simulink model "observe_bldc"  (R2020a)
settings: Solver=FixedStepDiscrete  StartTime=0.0  StopTime=10  FixedStep=50e-6  RelTol=1e-3
undefined symbols (not defined in the file): sigbuilder_block
libraries: nesl_utility x12, ee_lib x9, fl_lib x6, simulink x2
settings Model: Creator=Tinh_deptrai  LastModifiedBy=Tinh_deptrai
settings SolverCC: AlgebraicLoopSolver=LineSearch

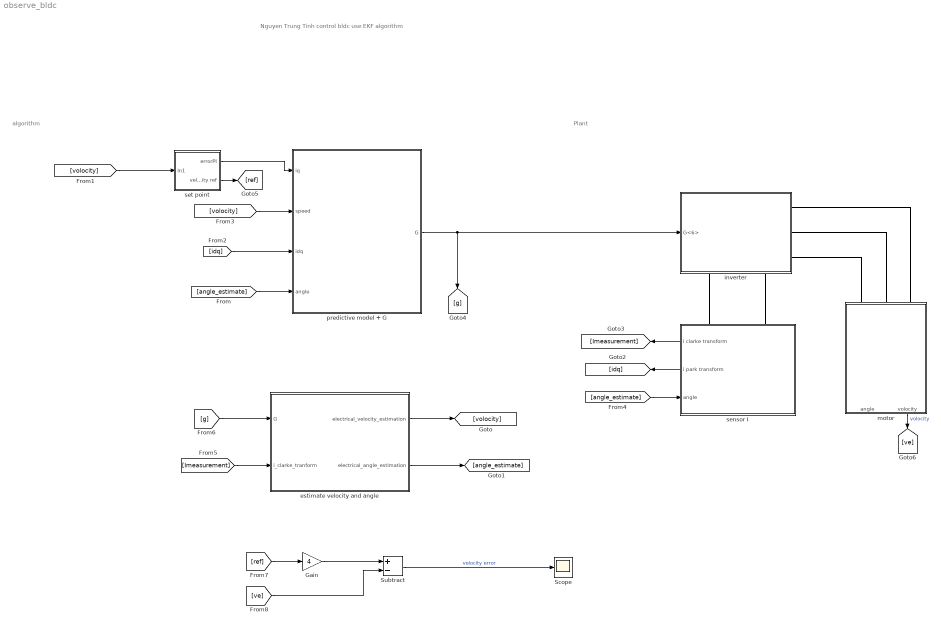
== system observe_bldc ==
  note: algorithm
  note: Nguyen Trung Tinh
      | control bldc use EKF algorithm
  note: Plant
  Gain : Gain  Gain=4
  Scope : Scope
  Subtract : Sum  Inputs=+-
  estimate velocity and angle : Subsystem
  inverter : Subsystem
      settings: PortSchema="{\"entries\":[{\"content\":{\"sides\":[{\"content\":{\"connectorIds\":[\"In1\"]},\"type\":\"ConnectorPlacement.EquallySpacedRectSide\",\"uuid\":\"9f8e1654-e76f-4ccd-87ff-712360a9448c\"},{\"content\":{\"connectorIds\":[\"RConn1\",\"RConn2\",\"RConn3\"],\"side\":\"RIGHT\"},\"type\":\"ConnectorPlacement.EquallySpacedRectSide\",\"uuid\":\"1603b82b-d8dc-4962-8b2e-607a69af6851\"},{\"content\":{\"connectorIds\":[],\"side\":\"TOP\"},\"type\":\"ConnectorPlacement.EquallySpacedRectSide\",\"uuid\":\"a55eb90c-eada-4bfc-8f9e-d2c70cbe25bd\"},{\"content\":{\"connectorIds\":[\"RConn4\",\"RConn5\"],\"side\":\"BOTTOM\"},\"type\":\"ConnectorPlacement.EquallySpacedRectSide\",\"uuid\":\"5facc57d-ea89-4f5b-8b06-1001d422b94e\"}]},\"type\":\"ConnectorPlacement.EquallySpacedConnector\",\"uuid\":\"acd0f578-42d7-4dc3-aef0-1ec9509de6cd\"}],\"packageUris\":[\"http://schema.mathworks.com/mf0/Connector/19700101\"],\"version\":\"1.0\"}"
  motor : Subsystem
  predictive model + G : Subsystem
  sensor I : Subsystem
      settings: PortSchema="{\"entries\":[{\"content\":{\"sides\":[{\"content\":{\"connectorIds\":[]},\"type\":\"ConnectorPlacement.EquallySpacedRectSide\",\"uuid\":\"0a592258-b95b-4330-8c63-2a9e4347ecac\"},{\"content\":{\"connectorIds\":[\"Out1\",\"Out2\",\"In1\"],\"side\":\"RIGHT\"},\"type\":\"ConnectorPlacement.EquallySpacedRectSide\",\"uuid\":\"44663962-0eca-4dc4-9145-5c0dbec9ec3a\"},{\"content\":{\"connectorIds\":[\"LConn1\",\"LConn2\"],\"side\":\"TOP\"},\"type\":\"ConnectorPlacement.EquallySpacedRectSide\",\"uuid\":\"ad629d0d-eb0f-4771-8bbd-1df9727b2b70\"}]},\"type\":\"ConnectorPlacement.EquallySpacedConnector\",\"uuid\":\"befa916a-8a4b-411d-a992-da4f8df3c86c\"}],\"packageUris\":[\"http://schema.mathworks.com/mf0/Connector/19700101\"],\"version\":\"1.0\"}"
  set point : Subsystem
  wires:
  [volocity] -> set point/1(In1)
  sensor I/1(" i clarke transform") -> [Imeasurement]
  sensor I/2(i park transform) -> [idq]
  set point/1(errorPI) -> predictive model + G/1(iq)
  [idq] -> predictive model + G/3(idq)
  [g] -> estimate velocity and angle/1(G)
  [Imeasurement] -> estimate velocity and angle/2(i_clarke_tranform)
  [angle_estimate] -> predictive model + G/4(angle)
  [volocity] -> predictive model + G/2(speed)
  [angle_estimate] -> sensor I/1(angle)
  predictive model + G/1(G) -> inverter/1(G<6>), [g]
  estimate velocity and angle/1(electrical_velocity_estimation) -> [volocity]
  estimate velocity and angle/2(electrical_angle_estimation) -> [angle_estimate]
  set point/2(velocity ref) -> [ref]
  [ref] -> Gain/1
  motor/2(volocity) -> [ve]  "volocity"
  [ve] -> Subtract/2
  Subtract/1 -> Scope/1  "velocity error"
  Gain/1 -> Subtract/1
  connections:
  motor/LConn1 -- inverter/RConn3
  motor/LConn2 -- inverter/RConn2
  motor/LConn3 -- inverter/RConn1
  sensor I/LConn2 -- inverter/RConn4
  sensor I/LConn1 -- inverter/RConn5

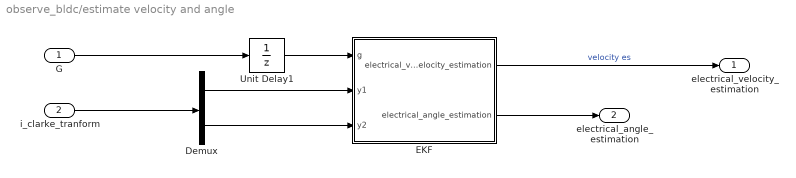
== system observe_bldc/estimate velocity and angle ==
  G : Inport
  i_clarke_tranform : Inport  Port=2
  Demux : Demux  Outputs=2
  EKF : Subsystem
  Unit Delay1 : UnitDelay  InitialCondition=1  SampleTime=-1  HasFrameUpgradeWarning=on
  electrical_velocity_estimation : Outport
  electrical_angle_estimation : Outport  Port=2
  wires:
  EKF/2(electrical_angle_estimation) -> electrical_angle_estimation/1
  Unit Delay1/1 -> EKF/1(g)
  i_clarke_tranform/1 -> Demux/1
  G/1 -> Unit Delay1/1
  Demux/1 -> EKF/2(y1)
  Demux/2 -> EKF/3(y2)
  EKF/1(electrical_velocity_estimation) -> electrical_velocity_estimation/1  "velocity es"

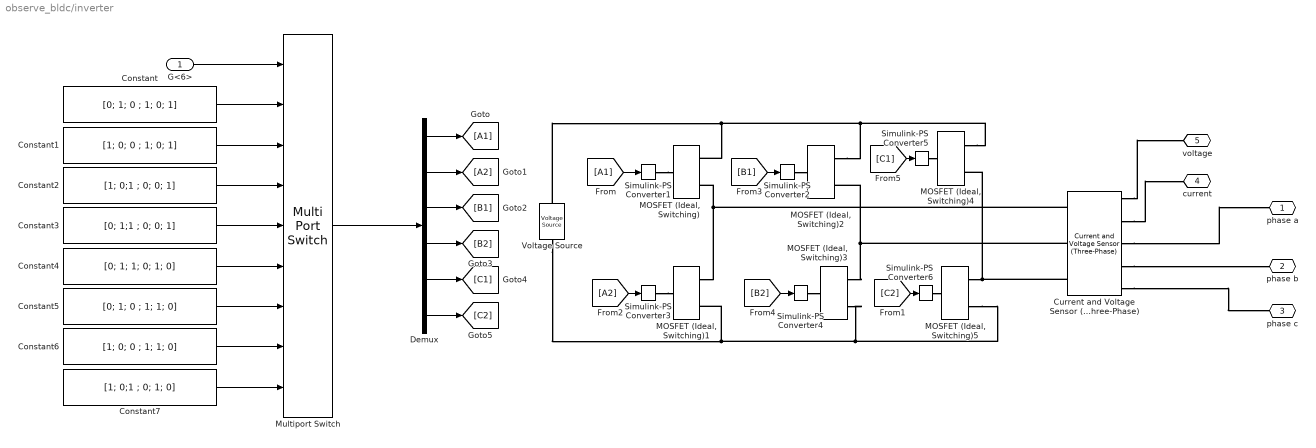
== system observe_bldc/inverter ==
  G<6> : Inport
  Constant : Constant  Value=[0; 1; 0 ; 1; 0; 1]
  Constant1 : Constant  Value=[1; 0; 0 ; 1; 0; 1]
  Constant2 : Constant  Value=[1; 0;1 ; 0; 0; 1]
  Constant3 : Constant  Value=[0; 1;1 ; 0; 0; 1]
  Constant4 : Constant  Value=[0; 1; 1; 0; 1; 0]
  Constant5 : Constant  Value=[0; 1; 0 ; 1; 1; 0]
  Constant6 : Constant  Value=[1; 0; 0 ; 1; 1; 0]
  Constant7 : Constant  Value=[1; 0;1 ; 0; 1; 0]
  Current and Voltage Sensor (Three-Phase) : ee_lib/Sensors & Transducers/Current and Voltage Sensor (Three-Phase)  vMeasurementType=ee.enum.vmeasurement.lg  outputUnit=ee.enum.unit.si  SRated=100e6 V*A  VRated=24e3 V  I_specify=off  I_priority=None  I=[ 0 0 0 ] A  I_nominal_specify=off  I_nominal_unit=A  I_nominal_value=1  V_specify=off  V_priority=None  V=[ 0 0 0 ] V  V_nominal_specify=off  V_nominal_unit=V  V_nominal_value=1
      settings: SourceProductBaseCode=PS  InternalSimscapePortConfiguration="{\"Bottom\":[],\"Left\":[{\"id\":\"a1\",\"label\":\"a1\",\"type\":\"foundation.electrical.electrical\"},{\"id\":\"b1\",\"label\":\"b1\",\"type\":\"foundation.electrical.electrical\"},{\"id\":\"c1\",\"label\":\"c1\",\"type\":\"foundation.electrical.electrical\"}],\"Right\":[{\"id\":\"V_output\",\"label\":\"V\",\"type\":\"output\"},{\"id\":\"I_output\",\"label\":\"I\",\"type\":\"output\"},{\"id\":\"a2\",\"label\":\"a2\",\"type\":\"foundation.electrical.electrical\"},{\"id\":\"b2\",\"label\":\"b2\",\"type\":\"foundation.electrical.electrical\"},{\"id\":\"c2\",\"label\":\"c2\",\"type\":\"foundation.electrical.electrical\"}],\"Top\":[]}"
  Demux : Demux  Outputs=6
  MOSFET (Ideal, Switching){,1..5} (6 alike) : ee_lib/Semiconductors & Converters/MOSFET (Ideal, Switching)  Rds=0.01 Ohm  Goff=1e-6 1/Ohm  Vth=0.5 V  diode_param=1  diode_Vf=0.8 V  diode_Ron=0.001 Ohm  diode_Goff=1e-5 1/Ohm  diode_C=50e-9 F  diode_iRM=-235 A  diode_iF=300 A  diode_idot=-50 A/us  diode_trr_param=1  diode_trr_factor=3  diode_trr=15 us  diode_Qrr=1500 s*uA  thermal_loss_option=2  Voff=300 V  Tau=1e-4 s  Tj=[298.15, 398.15] K  Iout_scalar=600 A  Eon_scalar=22.86e-3 J  Eoff_scalar=17.14e-3 J  Von_scalar=2.7 V  Iout_data=[0, 10, 50, 100, 200, 400, 600] A  Eon_data=[0, .29, 1.43, 2.86, 5.71, 13.14, 22.86; 0, .57, 2.63, 5.14, 10.29, 20.57, 30.29] * 1e-3 J  Eoff_data=[0, .21, 1.07, 2.14, 4.29, 9.86, 17.14; 0, .43, 1.97, 3.86, 7.71, 15.43, 22.71] * 1e-3 J  Von_data=[0, 1.1, 1.3, 1.45, 1.75, 2.25, 2.7; 0, 1, 1.15, 1.35, 1.7, 2.35, 3] V
  Multiport Switch : MultiPortSwitch  Inputs=8
  Simulink-PS Converter{1..6} (6 alike) : nesl_utility/Simulink-PS Converter  PhysicalDomain=network_engine_domain  SubClassName=ps_input  LeftPortType=input  RightPortType=output  PseudoPeriodic=off  Frequencies=[]  NoiseDistribution=none  NoiseParameters=[]  Unit=1  AffineConversion=off  FilteringAndDerivatives=provide  SimscapeFilterOrder=1  InputFilterTimeConstant=0.001  UdotUserProvided=0
  Voltage Source : ee_lib/Sources/Voltage Source  dc_voltage=48 V  ac_voltage=0 V  ac_shift=0 rad  ac_frequency=0 Hz  noise_mode=0  PSD=0 V^2/Hz  repeatability=1  auto_seed=4120125298  user_seed=0  sample_time=1e-3 s  i_specify=off  i_priority=None  i=0 A  i_nominal_specify=off  i_nominal_unit=A  i_nominal_value=1  v_specify=off  v_priority=None  v=0 V  v_nominal_specify=off  v_nominal_unit=V  v_nominal_value=1
  phase a : PMIOPort  Side=Right
  phase b : PMIOPort  Port=2  Side=Right
  phase c : PMIOPort  Port=3  Side=Right
  current : PMIOPort  Port=4  Side=Right
  voltage : PMIOPort  Port=5  Side=Right
  wires:
  Demux/4 -> [B2]
  Demux/1 -> [A1]
  [C2] -> Simulink-PS Converter6/1
  [A1] -> Simulink-PS Converter1/1
  Demux/3 -> [B1]
  [B1] -> Simulink-PS Converter2/1
  Demux/5 -> [C1]
  [A2] -> Simulink-PS Converter3/1
  Demux/2 -> [A2]
  Demux/6 -> [C2]
  [C1] -> Simulink-PS Converter5/1
  [B2] -> Simulink-PS Converter4/1
  G<6>/1 -> Multiport Switch/1
  Multiport Switch/1 -> Demux/1
  Constant/1 -> Multiport Switch/2
  Constant1/1 -> Multiport Switch/3
  Constant2/1 -> Multiport Switch/4
  Constant3/1 -> Multiport Switch/5
  Constant4/1 -> Multiport Switch/6
  Constant5/1 -> Multiport Switch/7
  Constant6/1 -> Multiport Switch/8
  Constant7/1 -> Multiport Switch/9
  connections:
  Voltage Source/RConn1 -- "MOSFET (Ideal, Switching)5"/RConn2 -- "MOSFET (Ideal, Switching)3"/RConn2 -- "MOSFET (Ideal, Switching)1"/RConn2
  Simulink-PS Converter5/RConn1 -- "MOSFET (Ideal, Switching)4"/LConn1
  Voltage Source/LConn1 -- "MOSFET (Ideal, Switching)4"/RConn1 -- "MOSFET (Ideal, Switching)2"/RConn1 -- "MOSFET (Ideal, Switching)"/RConn1
  Simulink-PS Converter2/RConn1 -- "MOSFET (Ideal, Switching)2"/LConn1
  "MOSFET (Ideal, Switching)1"/RConn1 -- Current and Voltage Sensor (Three-Phase)/LConn1 -- "MOSFET (Ideal, Switching)"/RConn2
  Simulink-PS Converter1/RConn1 -- "MOSFET (Ideal, Switching)"/LConn1
  Current and Voltage Sensor (Three-Phase)/RConn5 -- phase c/RConn1
  "MOSFET (Ideal, Switching)5"/RConn1 -- "MOSFET (Ideal, Switching)4"/RConn2 -- Current and Voltage Sensor (Three-Phase)/LConn3
  Current and Voltage Sensor (Three-Phase)/RConn4 -- phase b/RConn1
  Simulink-PS Converter4/RConn1 -- "MOSFET (Ideal, Switching)3"/LConn1
  "MOSFET (Ideal, Switching)3"/RConn1 -- "MOSFET (Ideal, Switching)2"/RConn2 -- Current and Voltage Sensor (Three-Phase)/LConn2
  Simulink-PS Converter6/RConn1 -- "MOSFET (Ideal, Switching)5"/LConn1
  Simulink-PS Converter3/RConn1 -- "MOSFET (Ideal, Switching)1"/LConn1
  Current and Voltage Sensor (Three-Phase)/RConn3 -- phase a/RConn1
  Current and Voltage Sensor (Three-Phase)/RConn1 -- voltage/RConn1
  Current and Voltage Sensor (Three-Phase)/RConn2 -- current/RConn1

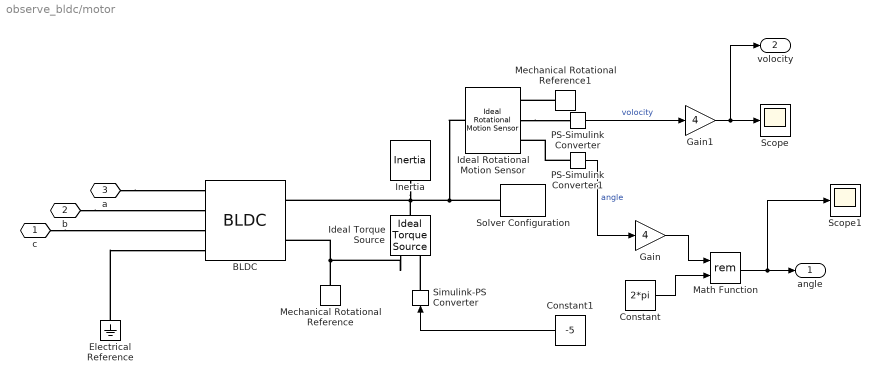
== system observe_bldc/motor ==
  BLDC : ee_lib/Electromechanical/Permanent Magnet/BLDC  winding_type=ee.enum.statorconnection.wye  rotor_param=1  pm_flux_linkage=0.175 Wb  theta_constant=pi / 12 rad  emf_max=9.6 V  DphiDtheta_tab=[0, -.1528, -.1528, .1528, .1528, 0] Wb/rad  back_emf_tab=[0, -9.6, -9.6, 9.6, 9.6, 0] V  rotor_angle_tab=[0, 7.5, 22.5, 37.5, 52.5, 60] deg  w_meas=600 rpm  nPolePairs=4  stator_param=ee.enum.statorparam.LsLmMs  machine_param=ee.enum.dqparameterization.constant  Ld=0.00022 H  Lq=0.00022 H  idVec=[-200, 0, 200] A  iqVec=[-200, 0, 200] A  LdMatrix=0.00022 * ones(3, 3) H  LqMatrix=0.00022 * ones(3, 3) H  L0=0.00016 H  Ls=8.5 mH  Lm=0.001 mH  Ms=0.02 mH  Rs=0.2 Ohm  zero_sequence=ee.enum.park.zerosequence.exclude  J=0.04 kg*m^2  lam=0 N*m/(rad/s)  axes_param=2  i_d_specify=off  i_d_priority=None  i_d=0 A  i_d_nominal_specify=off  i_d_nominal_unit=A  i_d_nominal_value=1  i_q_specify=off  i_q_priority=None  i_q=0 A  i_q_nominal_specify=off  i_q_nominal_unit=A  i_q_nominal_value=1  torque_specify=off  torque_priority=None  torque=0 N*m  torque_nominal_specify=off  torque_nominal_unit=N*m  torque_nominal_value=1  angular_velocity_specify=off  angular_velocity_priority=High  angular_velocity=0 rpm  angular_velocity_nominal_specify=off  angular_velocity_nominal_unit=rpm  angular_velocity_nominal_value=1  angular_position_specify=on  angular_position_priority=High  angular_position=90 deg  angular_position_nominal_specify=off  angular_position_nominal_unit=deg  angular_position_nominal_value=1  loss_param=ee.enum.ironloss.none  losses_oc=[0, 0, 0] W  losses_sc=[0, 0, 0] W  f_losses=60 Hz  Isc_losses=95 A  Tmeas=298.15 K  alpha=3.93e-3 1/K  alpha_flux=-0.001 1/K  stator_thermal_mass=100 J/K  rotor_thermal_mass=200 J/K  Rm_percent_rotor=90  Rd_percent_rotor=30  temperatureA_specify=off  temperatureA_priority=High  temperatureA=25 degC  temperatureA_nominal_specify=off  temperatureA_nominal_unit=degC  temperatureA_nominal_value=1  temperatureB_specify=off  temperatureB_priority=High  temperatureB=25 degC  temperatureB_nominal_specify=off  temperatureB_nominal_unit=degC  temperatureB_nominal_value=1  temperatureC_specify=off  temperatureC_priority=High  temperatureC=25 degC  temperatureC_nominal_specify=off  temperatureC_nominal_unit=degC  temperatureC_nominal_value=1  temperatureR_specify=off  temperatureR_priority=High  temperatureR=25 degC  temperatureR_nominal_specify=off  temperatureR_nominal_unit=degC  temperatureR_nominal_value=1
      settings: SourceProductBaseCode=PS  InternalSimscapePortConfiguration="{\"Bottom\":[],\"Left\":[{\"id\":\"a\",\"label\":\"a\",\"type\":\"foundation.electrical.electrical\"},{\"id\":\"b\",\"label\":\"b\",\"type\":\"foundation.electrical.electrical\"},{\"id\":\"c\",\"label\":\"c\",\"type\":\"foundation.electrical.electrical\"},{\"id\":\"n\",\"label\":\"n\",\"type\":\"foundation.electrical.electrical\"}],\"Right\":[{\"id\":\"R\",\"label\":\"R\",\"type\":\"foundation.mechanical.rotational.rotational\"},{\"id\":\"C\",\"label\":\"C\",\"type\":\"foundation.mechanical.rotational.rotational\"}],\"Top\":[]}"
  Constant : Constant  Value=2*pi
  Constant1 : Constant  Value=-5
  Electrical Reference : fl_lib/Electrical/Electrical Elements/Electrical Reference
  Gain : Gain  Gain=4
  Gain1 : Gain  Gain=4
  Ideal Rotational Motion Sensor : fl_lib/Mechanical/Mechanical Sensors/Ideal Rotational Motion Sensor  wrap_angle=simscape.enum.onoff.off  offset=0 rad
  Ideal Torque Source : fl_lib/Mechanical/Mechanical Sources/Ideal Torque Source
  Inertia : fl_lib/Mechanical/Rotational Elements/Inertia  inertia=0.01 kg*m^2  w_specify=off  w_priority=High  w=0 rad/s  w_nominal_specify=off  w_nominal_unit=rad/s  w_nominal_value=1  t_specify=off  t_priority=None  t=0 N*m  t_nominal_specify=off  t_nominal_unit=N*m  t_nominal_value=1
  Math Function : Math  Operator=rem  SaturateOnIntegerOverflow=on
  Mechanical Rotational Reference : fl_lib/Mechanical/Rotational Elements/Mechanical Rotational Reference
  Mechanical Rotational Reference1 : fl_lib/Mechanical/Rotational Elements/Mechanical Rotational Reference
  PS-Simulink Converter : nesl_utility/PS-Simulink Converter  PhysicalDomain=network_engine_domain  SubClassName=ps_output  LeftPortType=input  RightPortType=output  PseudoPeriodic=off  Frequencies=[]  Unit=rad/s  AffineConversion=off
  PS-Simulink Converter1 : nesl_utility/PS-Simulink Converter  PhysicalDomain=network_engine_domain  SubClassName=ps_output  LeftPortType=input  RightPortType=output  PseudoPeriodic=off  Frequencies=[]  Unit=rad  AffineConversion=off
  Scope : Scope
  Scope1 : Scope
  Simulink-PS Converter : nesl_utility/Simulink-PS Converter  PhysicalDomain=network_engine_domain  SubClassName=ps_input  LeftPortType=input  RightPortType=output  PseudoPeriodic=off  Frequencies=[]  NoiseDistribution=none  NoiseParameters=[]  Unit=1  AffineConversion=off  FilteringAndDerivatives=provide  SimscapeFilterOrder=1  InputFilterTimeConstant=0.001  UdotUserProvided=0
  Solver Configuration : nesl_utility/Solver Configuration  PhysicalDomain=network_engine_domain  SubClassName=solver  LeftPortType=input  RightPortType=generic  Tones=[]  Harmonics=[]  SimulateNoise=off  Profile=off  UseLocalSampling=off  EnableSwitchedLinearOptims=on  FrequencyDomain=off  UseCCode=off  RelTol=0.001  AbsTol=1e-06  MinStep=1e-09  ToWorkspace=off  RevertToSquareIcSolve=off  NumHomotopyIterations=100  PhasorMode=off  PhasorModeNumHarmonics=1  DoDC=off  ResidualTolerance=1e-9  UseLocalSolver=on  LocalSolverChoice=NE_BACKWARD_EULER_ADVANCER  LocalSolverSampleTime=50e-6  DoFixedCost=on  MaxNonlinIter=3  MaxModeIter=2  LinearAlgebra=auto  EquationFormulation=NE_TIME_EF  DelaysMemoryBudget=1024  AutomaticFiltering=on  FilteringTimeConstant=0.001  PartitionStorageMethod=AS_NEEDED  PartitionMemoryBudget=1024  PartitionMethod=ROBUST
  c : PMIOPort  Side=Left
  b : PMIOPort  Port=2  Side=Left
  a : PMIOPort  Port=3  Side=Left
  angle : Outport
  volocity : Outport  Port=2
  wires:
  PS-Simulink Converter/1 -> Gain1/1  "volocity"
  PS-Simulink Converter1/1 -> Gain/1  "angle"
  Math Function/1 -> Scope1/1, angle/1
  Constant/1 -> Math Function/2
  Gain1/1 -> volocity/1, Scope/1
  Gain/1 -> Math Function/1
  Constant1/1 -> Simulink-PS Converter/1
  connections:
  Ideal Rotational Motion Sensor/RConn2 -- PS-Simulink Converter/LConn1
  Solver Configuration/RConn1 -- Ideal Rotational Motion Sensor/LConn1 -- BLDC/RConn1 -- Inertia/LConn1 -- Ideal Torque Source/LConn1
  Mechanical Rotational Reference/LConn1 -- Ideal Torque Source/RConn2 -- BLDC/RConn2
  a/RConn1 -- BLDC/LConn1
  Electrical Reference/LConn1 -- BLDC/LConn4
  Mechanical Rotational Reference1/LConn1 -- Ideal Rotational Motion Sensor/RConn1
  PS-Simulink Converter1/LConn1 -- Ideal Rotational Motion Sensor/RConn3
  b/RConn1 -- BLDC/LConn2
  c/RConn1 -- BLDC/LConn3
  Simulink-PS Converter/RConn1 -- Ideal Torque Source/RConn1

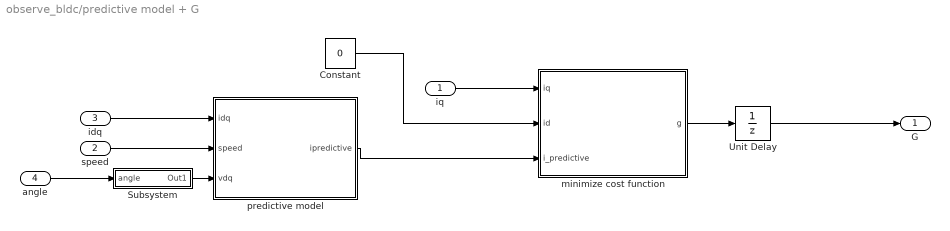
== system observe_bldc/predictive model + G ==
  iq : Inport
  speed : Inport  Port=2
  idq : Inport  Port=3
  angle : Inport  Port=4
  Constant : Constant  Value=0
  Subsystem : Subsystem
  Unit Delay : UnitDelay  InitialCondition=1  SampleTime=-1  HasFrameUpgradeWarning=on
  minimize cost function : MATLAB Function  TreatAsAtomicUnit=on
  predictive model : MATLAB Function  TreatAsAtomicUnit=on
  G : Outport
  wires:
  speed/1 -> predictive model/2(speed)
  minimize cost function/1(g) -> Unit Delay/1
  idq/1 -> predictive model/1(idq)
  predictive model/1(ipredictive) -> minimize cost function/3(i_predictive)
  Unit Delay/1 -> G/1
  iq/1 -> minimize cost function/1(iq)
  Subsystem/1(Out1) -> predictive model/3(vdq)
  angle/1 -> Subsystem/1(angle)
  Constant/1 -> minimize cost function/2(id)

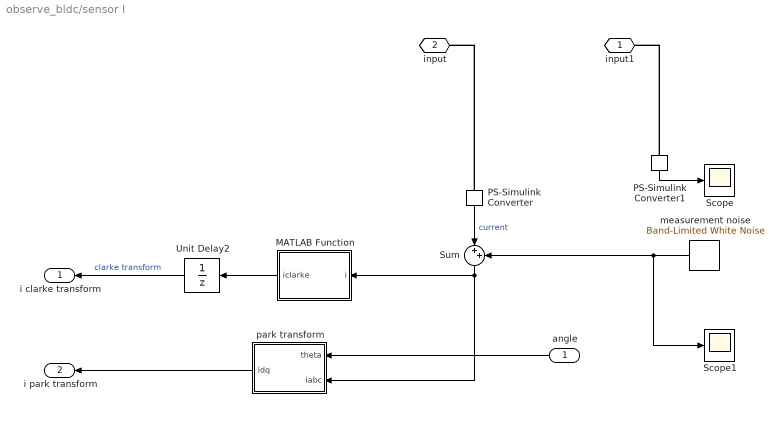
== system observe_bldc/sensor I ==
  angle : Inport
  MATLAB Function : MATLAB Function  TreatAsAtomicUnit=on
  PS-Simulink Converter : nesl_utility/PS-Simulink Converter  PhysicalDomain=network_engine_domain  SubClassName=ps_output  LeftPortType=input  RightPortType=output  PseudoPeriodic=off  Frequencies=[]  Unit=A  AffineConversion=off
  PS-Simulink Converter1 : nesl_utility/PS-Simulink Converter  PhysicalDomain=network_engine_domain  SubClassName=ps_output  LeftPortType=input  RightPortType=output  PseudoPeriodic=off  Frequencies=[]  Unit=V  AffineConversion=off
  Scope : Scope
  Scope1 : Scope
  Sum : Sum  Inputs=|++
  Unit Delay2 : UnitDelay  SampleTime=-1  HasFrameUpgradeWarning=on
  measurement noise : simulink/Sources/Band-Limited White Noise  Cov=[0.01*50e-6]  Ts=50e-6  seed=[23341]
  park transform : MATLAB Function  TreatAsAtomicUnit=on
  input1 : PMIOPort  Side=Left
  input : PMIOPort  Port=2  Side=Left
  " i clarke transform" : Outport
  i park transform : Outport  Port=2
  wires:
  Unit Delay2/1 -> " i clarke transform"/1  "clarke transform"
  PS-Simulink Converter1/1 -> Scope/1
  MATLAB Function/1(iclarke) -> Unit Delay2/1
  park transform/1(idq) -> i park transform/1
  angle/1 -> park transform/1(theta)
  PS-Simulink Converter/1 -> Sum/1  "current"
  Sum/1 -> park transform/2(iabc), MATLAB Function/1(i)
  measurement noise/1 -> Scope1/1, Sum/2
  connections:
  PS-Simulink Converter/LConn1 -- input/RConn1
  PS-Simulink Converter1/LConn1 -- input1/RConn1

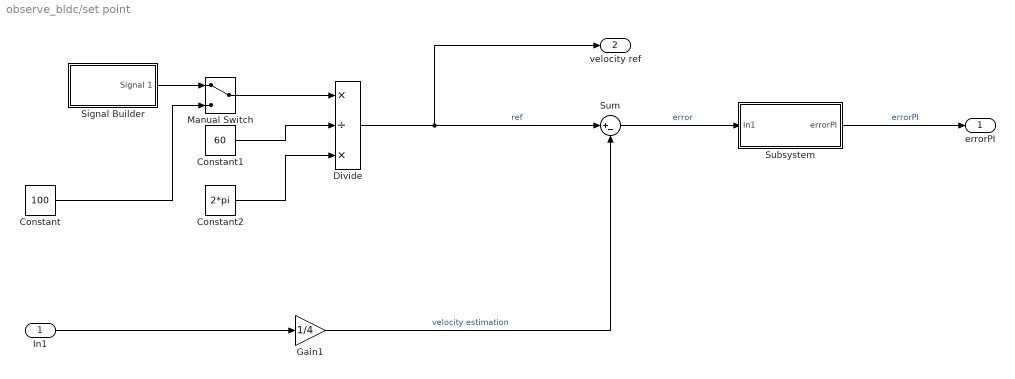
== system observe_bldc/set point ==
  In1 : Inport
  Constant : Constant  Value=100
  Constant1 : Constant  Value=60
  Constant2 : Constant  Value=2*pi
  Divide : Product  Inputs=*/*
  Gain1 : Gain  Gain=1/4
  Manual Switch : ManualSwitch
  Signal Builder : Subsystem  Tag=STV Subsys  LoadFcn=sigbuilder_block('load');  StartFcn=sigbuilder_block('start');  StopFcn=sigbuilder_block('stop');  ClipboardFcn=sigbuilder_block('clipboard');  mask(Sigbuilder block){tuvar=[0:10]}
      mask help: Simulink:masks:SigbuilderBlock_MD
      mask init:
      | if ~strcmp(get_param(bdroot(gcbh),'SimulationStatus'),'stopped') tuvar = sigbuilder_block('maskInit'); end
      settings: CopyFcn=sigbuilder_block('copy');  DeleteFcn=sigbuilder_block('delete');  ModelCloseFcn=sigbuilder_block('modelClose');  PreSaveFcn=sigbuilder_block('preSave');  PauseFcn=sigbuilder_block('pause');  ContinueFcn=sigbuilder_block('continue');  NameChangeFcn=sigbuilder_block('namechange');  OpenFcn=sigbuilder_block('open',[5.4 30 1141.2 522.6 ]);  CloseFcn=sigbuilder_block('close');
      mask Display: plot(0, 0, 100, 100,[2, 2, 32, 32, 2], [68, 8, 8, 68, 68],[32, 2], [38, 38], [32, 19, 2],[53, 60, 44], [32, 17, 17, 2],[16, 16, 31, 31]);txt = getActiveGroup(gcbh);text(2, 100, txt,'verticalAlignment', 'top');
  Subsystem : Subsystem  mask{Kp=1.05, Ki=0.001/1.05}
  Sum : Sum  Inputs=|+-
  errorPI : Outport
  velocity ref : Outport  Port=2
  wires:
  Gain1/1 -> Sum/2  "velocity estimation"
  Sum/1 -> Subsystem/1(In1)  "error"
  Constant/1 -> Manual Switch/2
  Subsystem/1(errorPI) -> errorPI/1  "errorPI"
  Signal Builder/1(Signal 1) -> Manual Switch/1
  In1/1 -> Gain1/1
  Manual Switch/1 -> Divide/1
  Divide/1 -> velocity ref/1, Sum/1  "ref"
  Constant1/1 -> Divide/2
  Constant2/1 -> Divide/3

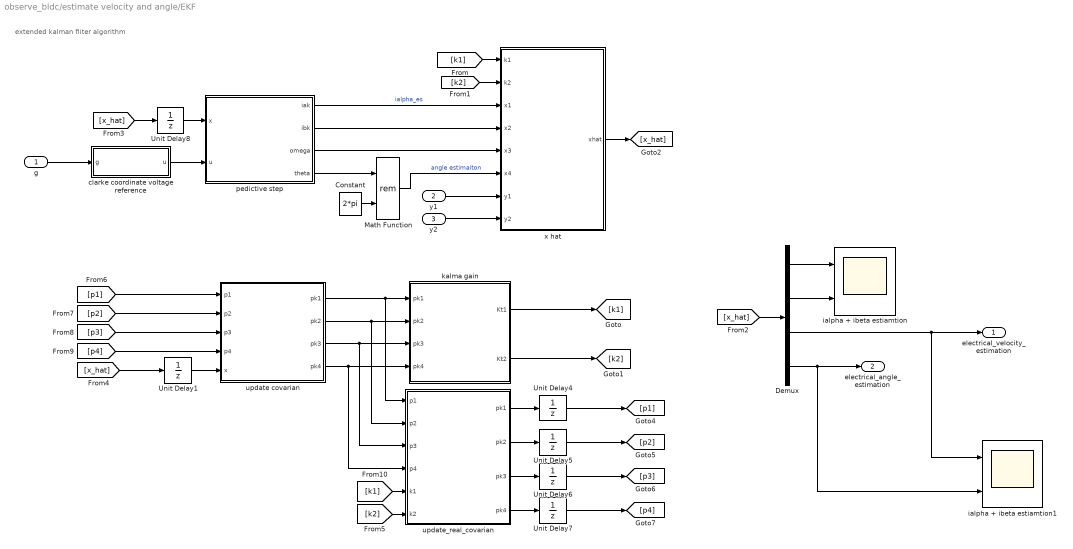
== system observe_bldc/estimate velocity and angle/EKF ==
  note: extended kalman fliter algorithm
  g : Inport
  y1 : Inport  Port=2
  y2 : Inport  Port=3
  Constant : Constant  Value=2*pi
  Demux : Demux
  Math Function : Math  Operator=rem  SaturateOnIntegerOverflow=on
  Unit Delay1 : UnitDelay  InitialCondition=[0 0 0 0]  SampleTime=-1  HasFrameUpgradeWarning=on
  Unit Delay4 : UnitDelay  InitialCondition=[0.1;0;0;0]  SampleTime=-1  HasFrameUpgradeWarning=on
  Unit Delay5 : UnitDelay  InitialCondition=[0; 0.2; 0; 0]  SampleTime=-1  HasFrameUpgradeWarning=on
  Unit Delay6 : UnitDelay  InitialCondition=[0;0;0.5;0]  SampleTime=-1  HasFrameUpgradeWarning=on
  Unit Delay7 : UnitDelay  InitialCondition=[0;0;0;0.02]  SampleTime=-1  HasFrameUpgradeWarning=on
  Unit Delay8 : UnitDelay  InitialCondition=[0 0 0 0.01]  SampleTime=-1  HasFrameUpgradeWarning=on
  clarke coordinate voltage reference : Subsystem
  ialpha + ibeta estiamtion : Scope  NumInputPorts=2
  ialpha + ibeta estiamtion1 : Scope  NumInputPorts=2
  kalma gain : MATLAB Function  TreatAsAtomicUnit=on
  pedictive step : MATLAB Function  TreatAsAtomicUnit=on
  update covarian : MATLAB Function  TreatAsAtomicUnit=on
  update_real_covarian : MATLAB Function  TreatAsAtomicUnit=on
  x hat : MATLAB Function  TreatAsAtomicUnit=on
  electrical_velocity_estimation : Outport
  electrical_angle_estimation : Outport  Port=2
  wires:
  g/1 -> clarke coordinate voltage reference/1(g)
  clarke coordinate voltage reference/1(u) -> pedictive step/2(u)
  update covarian/1(pk1) -> update_real_covarian/1(p1), kalma gain/1(pk1)
  update covarian/2(pk2) -> update_real_covarian/2(p2), kalma gain/2(pk2)
  update covarian/3(pk3) -> kalma gain/3(pk3), update_real_covarian/3(p3)
  update covarian/4(pk4) -> kalma gain/4(pk4), update_real_covarian/4(p4)
  pedictive step/1(iak) -> x hat/3(x1)  "ialpha_es"
  pedictive step/2(ibk) -> x hat/4(x2)
  y1/1 -> x hat/7(y1)
  y2/1 -> x hat/8(y2)
  kalma gain/1(Kt1) -> [k1]
  kalma gain/2(Kt2) -> [k2]
  [k1] -> x hat/1(k1)
  [k2] -> x hat/2(k2)
  update_real_covarian/1(pk1) -> Unit Delay4/1
  update_real_covarian/2(pk2) -> Unit Delay5/1
  update_real_covarian/3(pk3) -> Unit Delay6/1
  update_real_covarian/4(pk4) -> Unit Delay7/1
  [p1] -> update covarian/1(p1)
  [p2] -> update covarian/2(p2)
  [p3] -> update covarian/3(p3)
  [p4] -> update covarian/4(p4)
  Unit Delay4/1 -> [p1]
  Unit Delay5/1 -> [p2]
  Unit Delay6/1 -> [p3]
  Unit Delay7/1 -> [p4]
  pedictive step/3(omega) -> x hat/5(x3)
  pedictive step/4(theta) -> Math Function/1
  Math Function/1 -> x hat/6(x4)  "angle estimaiton"
  Constant/1 -> Math Function/2
  Demux/3 -> electrical_velocity_estimation/1, ialpha + ibeta estiamtion1/1
  Demux/1 -> ialpha + ibeta estiamtion/1
  Demux/2 -> ialpha + ibeta estiamtion/2
  x hat/1(xhat) -> [x_hat]
  [x_hat] -> Demux/1
  Unit Delay8/1 -> pedictive step/1(x)
  [x_hat] -> Unit Delay8/1
  Unit Delay1/1 -> update covarian/5(x)
  [x_hat] -> Unit Delay1/1
  [k1] -> update_real_covarian/5(k1)
  [k2] -> update_real_covarian/6(k2)
  Demux/4 -> ialpha + ibeta estiamtion1/2, electrical_angle_estimation/1

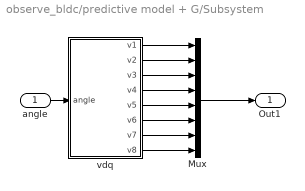
== system observe_bldc/predictive model + G/Subsystem ==
  angle : Inport
  Mux : Mux  Inputs=8
  vdq : MATLAB Function  TreatAsAtomicUnit=on
  Out1 : Outport
  wires:
  angle/1 -> vdq/1(angle)
  vdq/2(v2) -> Mux/2
  vdq/5(v5) -> Mux/5
  vdq/3(v3) -> Mux/3
  vdq/6(v6) -> Mux/6
  vdq/7(v7) -> Mux/7
  vdq/4(v4) -> Mux/4
  vdq/8(v8) -> Mux/8
  vdq/1(v1) -> Mux/1
  Mux/1 -> Out1/1

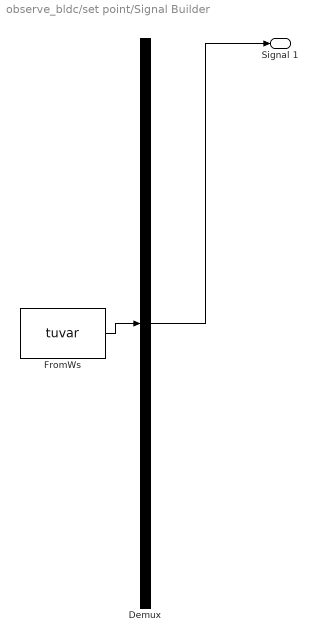
== system observe_bldc/set point/Signal Builder ==
  Demux : Demux  Tag=STV Demux  Outputs=1
      settings: DisplayOption=none
  FromWs : FromWorkspace  Tag=STV FromWs  VariableName=tuvar
      SigBuilderData=|
      | common.afterFinalStr = 'Extrapolate'
      | common.sampleTime = 0
      | dataSet.timeRange = [0 10]
      | dataSet.name = 'Group 1'
      | sbobj.Groups.Name = 'Group 1'
      | sbobj.Groups.Signals.Name = 'Signal 1'
      | sbobj.Groups.Signals.XData = [0 0.28 1.12 1.81 3.49 3.56 4.99 10]
      | sbobj.Groups.Signals.YData = [0 119 118 349 349 118 -20 -19]
  Signal 1 : Outport  Tag=STV Outport
  wires:
  Demux/1 -> Signal 1/1
  FromWs/1 -> Demux/1

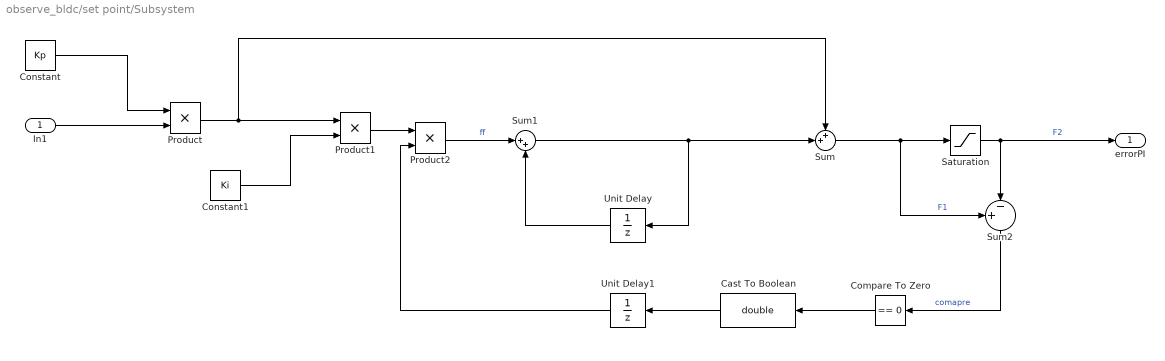
== system observe_bldc/set point/Subsystem ==
  In1 : Inport
  Cast To Boolean : DataTypeConversion  OutDataTypeStr=double
  Compare To Zero : simulink/Logic and Bit Operations/Compare To Zero  relop===  OutDataTypeStr=uint8
  Constant : Constant  Value=Kp
  Constant1 : Constant  Value=Ki
  Product : Product
  Product1 : Product
  Product2 : Product
  Saturation : Saturate  UpperLimit=10  LowerLimit=-10  LinearizeAsGain=off
  Sum : Sum  Inputs=++|
  Sum1 : Sum  Inputs=|++
  Sum2 : Sum  Inputs=+-|
  Unit Delay : UnitDelay  SampleTime=-1  HasFrameUpgradeWarning=on
  Unit Delay1 : UnitDelay  InitialCondition=1  SampleTime=-1  HasFrameUpgradeWarning=on
  errorPI : Outport
  wires:
  In1/1 -> Product/2
  Constant/1 -> Product/1
  Product/1 -> Product1/1, Sum/1
  Product1/1 -> Product2/1
  Constant1/1 -> Product1/2
  Product2/1 -> Sum1/1  "ff"
  Unit Delay/1 -> Sum1/2
  Sum1/1 -> Sum/2, Unit Delay/1
  Sum/1 -> Sum2/1, Saturation/1  "F1"
  Saturation/1 -> Sum2/2, errorPI/1  "F2"
  Sum2/1 -> Compare To Zero/1  "comapre"
  Compare To Zero/1 -> Cast To Boolean/1
  Unit Delay1/1 -> Product2/2
  Cast To Boolean/1 -> Unit Delay1/1

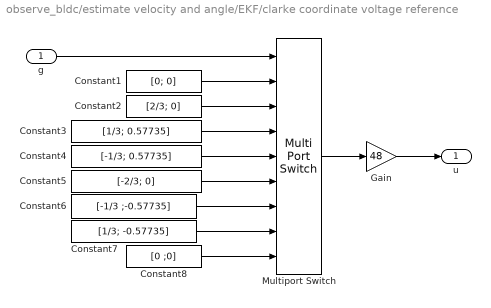
== system observe_bldc/estimate velocity and angle/EKF/clarke coordinate voltage reference ==
  g : Inport
  Constant1 : Constant  Value=[0; 0]
  Constant2 : Constant  Value=[2/3; 0]
  Constant3 : Constant  Value=[1/3; 0.57735]
  Constant4 : Constant  Value=[-1/3; 0.57735]
  Constant5 : Constant  Value=[-2/3; 0]
  Constant6 : Constant  Value=[-1/3 ;-0.57735]
  Constant7 : Constant  Value=[1/3; -0.57735]
  Constant8 : Constant  Value=[0 ;0]
  Gain : Gain  Gain=48
  Multiport Switch : MultiPortSwitch  Inputs=8
  u : Outport
  wires:
  Constant3/1 -> Multiport Switch/4
  Constant2/1 -> Multiport Switch/3
  Constant6/1 -> Multiport Switch/7
  Constant4/1 -> Multiport Switch/5
  Constant1/1 -> Multiport Switch/2
  Constant8/1 -> Multiport Switch/9
  Constant5/1 -> Multiport Switch/6
  Multiport Switch/1 -> Gain/1
  Constant7/1 -> Multiport Switch/8
  g/1 -> Multiport Switch/1
  Gain/1 -> u/1

== matlab function observe_bldc/estimate velocity and angle/EKF/update_real_covarian ==
  data: p1 input; pk1 output size=4; p2 input; p3 input; p4 input; k1 input; k2 input; pk2 output size=4; pk3 output size=4; pk4 output size=4
function [pk1,pk2,pk3,pk4] = fcn(p1, p2, p3, p4, k1, k2)
Ht = [1 0 0 0 ;
    0 1 0 0 ];
P = [p1 p2 p3 p4];
Kt = [k1 k2];

Pt=(eye(4) - Kt*Ht)*P;
pk1 = Pt(:,1);
pk2 = Pt(:,2);
pk3 = Pt(:,3);
pk4 = Pt(:,4);

== matlab function observe_bldc/sensor I/MATLAB Function ==
  data: i input; iclarke output
function iclarke = fcn(i)
ia = i(1,1);
ib = 1/sqrt(3)*(i(1,1) + 2*i(2,1));
iclarke = [ia;ib];

== matlab function observe_bldc/predictive model + G/predictive model ==
  data: idq input size=2; ipredictive output size=16; speed input size=1; vdq input
function ipredictive = fcn(idq, speed, vdq)
% phuong trinh cua dong co PMSM trong dq coordinate
% isd(k + 1) = (1 - Rs*Ts/Ls)*isd(k) + Ts*speed*isq(k) + Ts/Ls*vsd;
% isq(k + 1) = (1 - Rs*Ts/Ls)*isq(k) - Ts*speed*isd(k) + Ts/Ls*vsq;
% isd(k + 1) = A*isd(k) + B*isq(k) + C*vsd;
% isq(k + 1) = A*isq(k) - B*isd(k) + C*vsq;
%% bang chuyen doi v san qd
A = (1 - 0.2*50e-6/8.5e-3);
B = 50e-6*speed;
C = 50e-6/8.5e-3;
isd1 = A*idq(1,1) + B*idq(2,1) + C*vdq(1,1);
isq1 = A*idq(2,1) - B*idq(1,1) + C*vdq(2,1);
%
isd2 = A*idq(1,1) + B*idq(2,1) + C*vdq(3,1);
isq2 = A*idq(2,1) - B*idq(1,1) + C*vdq(4,1);
%
isd3 = A*idq(1,1) + B*idq(2,1) + C*vdq(5,1);
isq3 = A*idq(2,1) - B*idq(1,1) + C*vdq(6,1);
%
isd4 = A*idq(1,1) + B*idq(2,1) + C*vdq(7,1);
isq4 = A*idq(2,1) - B*idq(1,1) + C*vdq(8,1);
%
isd5 = A*idq(1,1) + B*idq(2,1) + C*vdq(9,1);
isq5 = A*idq(2,1) - B*idq(1,1) + C*vdq(10,1);
%
isd6 = A*idq(1,1) + B*idq(2,1) + C*vdq(11,1);
isq6 = A*idq(2,1) - B*idq(1,1) + C*vdq(12,1);
%
isd7 = A*idq(1,1) + B*idq(2,1) + C*vdq(13,1);
isq7 = A*idq(2,1) - B*idq(1,1) + C*vdq(14,1);
%
isd8 = A*idq(1,1) + B*idq(2,1) + C*vdq(15,1);
isq8 = A*idq(2,1) - B*idq(1,1) + C*vdq(16,1);

ipredictive = [isq1; isd1; isq2; isd2; isq3; isd3; isq4; isd4;
               isq5; isd5; isq6; isd6; isq7; isd7; isq8; isd8];

== matlab function observe_bldc/predictive model + G/minimize cost function ==
  data: iq input; id input; g output size=1; i_predictive input size=16
function g = fcn( iq,id, i_predictive)
gopt = inf ;
xopt = 1;
for i = 1:8
    if (i_predictive(2*i,1) > 15)
        l = inf;
    elseif ( i_predictive(2*i-1,1) > 15)
        l = inf;
    else 
        l = (iq - i_predictive(2*i-1,1))^2 + (id -i_predictive(2*i,1))^2;
    end
        if( l < gopt)
            gopt = l;
            xopt = i;          
        end
end
g = xopt;

== matlab function observe_bldc/sensor I/park transform ==
  data: theta input; idq output; iabc input
function idq = fcn(theta,iabc)
K = [cos(theta) cos(theta - 2*pi/3) cos(theta + 2*pi/3);
    -sin(theta) -sin(theta - 2*pi/3) -sin(theta + 2*pi/3)];
idq = K*iabc;

== matlab function observe_bldc/estimate velocity and angle/EKF/update covarian ==
  data: p1 input; pk1 output; p2 input; p3 input; p4 input; pk2 output; pk3 output; pk4 output; x input
function [pk1, pk2, pk3, pk4] = fcn(p1,p2,p3,p4, x)
ptemp = [p1  p2  p3  p4];
Rs = 0.2;
Ls = 8.5e-3;
Ts = 50e-6;
flux = 0.175;
Q = [0.2 0 0 0;
     0  0.2 0 0;
     0 0 1 0;
     0 0 0 0.001];
F = [1-Rs*Ts/Ls 0 flux*Ts*sin(x(4,1))/Ls flux*Ts*cos(x(4,1))*x(3,1)/Ls;
    0 1-Rs*Ts/Ls -flux*cos(x(4,1))*Ts/Ls flux*Ts*x(3,1)*sin(x(4,1))/Ls;
    0 0 1 0;
    0 0 Ts 1  ];
p = F*ptemp*F' + Q;
pk1 = p(:,1);
pk2 = p(:,2);
pk3 = p(:,3);
pk4 = p(:,4);

== matlab function observe_bldc/estimate velocity and angle/EKF/kalma gain ==
  data: pk1 input; Kt1 output size=4; pk2 input; pk3 input; pk4 input; Kt2 output size=4
function [Kt1,Kt2] = fcn(pk1,pk2,pk3,pk4)
Pt = [pk1  pk2  pk3 pk4];
Ht = [1 0 0 0 ;
    0 1 0 0 ];
Rt = [0.1 0
    0 0.1];

Kt = Pt*Ht'/(Ht*Pt*Ht' + Rt);
Kt1 = Kt(:,1);
Kt2 = Kt(:,2);

== matlab function observe_bldc/estimate velocity and angle/EKF/pedictive step ==
  data: x input; iak output; u input; ibk output; omega output; theta output
function [iak, ibk, omega, theta] = fcn(x,u)
Rs = 0.2;
Ls = 8.5e-3;
Ts =50e-6;
flux = 0.175;
iak = x(1,1)*(1-Rs*Ts/Ls) + Ts*flux*x(3,1)*sin(x(4,1))/Ls + Ts*u(1,1)/Ls;
ibk = x(2,1)*(1-Rs*Ts/Ls) - Ts*flux*x(3,1)*cos(x(4,1))/Ls + Ts*u(2,1)/Ls;
omega = x(3,1);
theta = x(4,1) + Ts*x(3,1);

== matlab function observe_bldc/estimate velocity and angle/EKF/x hat ==
  data: k1 input; xhat output size=4; k2 input; x1 input; x2 input; x3 input; x4 input; y1 input; y2 input
function xhat = fcn(k1, k2,x1, x2, x3,x4,y1,y2)
Kt = [k1 k2];
x = [x1;x2;x3;x4];
y = [y1;y2];
xm = [x1;x2];

xhat = x + Kt*(y-xm);

== matlab function observe_bldc/predictive model + G/Subsystem/vdq ==
  data: angle input; v1 output; v2 output; v3 output; v4 output; v5 output; v6 output; v7 output; v8 output
function [v1, v2, v3, v4, v5, v6, v7, v8] = fcn(angle)
Kp = 48*[ cos(angle) sin(angle) ;
       -sin(angle) cos(angle)];
v1 = Kp*[0 ; 0];
v2 = Kp*[2/3 ; 0];
v3 = Kp*[1/3; sqrt(3)/3];
v4 = Kp*[-1/3; sqrt(3)/3];
v5 = Kp*[-2/3; 0];
v6 = Kp*[-1/3; -sqrt(3)/3];
v7 = Kp*[ 1/3; -sqrt(3)/3];
v8 = Kp*[0; 0];
